simulink model "ADMIRE"  (R2021b)
settings: Solver=ode4  StartTime=0.0  StopTime=100  FixedStep=1e-2  RelTol=1e-3
undefined symbols (not defined in the file or in its folder): admireDB, Earth, WGS84
libraries: simulink_extras x112, simulink x27, aerolibutil x4, dspsigops x4, aerolibfltsims x3, sharedtransform x2, aerolibtransform2 x2, aerolibatmos2 x1, matrix_library x1, sharedutil x1, aerolibanimutils x1, vrlib x1
(part 10 of 15)

== system ADMIRE/Aircraft/Aerodynamics/CentripetalForceCoefficient/MachRegion2/Ccrbeta/Ccrbeta_ ==
  angleOfSideslip_deg : Inport
  angleOfAttack_deg : Inport  Port=2
  tflow : Inport  Port=3
  rc : Inport  Port=4
  Abs : Abs
  CCRBA_BETA_ALFA : Lookup_n-D  BreakpointsForDimension1=admireDB.aerodata_asym_ext.CCRBA.breakpoints.ALFA  BreakpointsForDimension2=admireDB.aerodata_asym_ext.CCRBA.breakpoints.BETA  BreakpointsForDimension3=[5, 7]  Table=admireDB.aerodata_asym_ext.CCRBA.newTable  ExtrapMethod=Clip  InternalRulePriority=Speed  RndMeth=Simplest  InputSameDT=on
      settings: InputPortMap=u0,u1
  Product : Product  Inputs=3
  Ccrbeta : Outport
  wires:
  Product/1 -> Ccrbeta/1
  rc/1 -> Product/3
  Abs/1 -> CCRBA_BETA_ALFA/2
  angleOfSideslip_deg/1 -> Abs/1
  angleOfAttack_deg/1 -> CCRBA_BETA_ALFA/1
  tflow/1 -> Product/2
  CCRBA_BETA_ALFA/1 -> Product/1

== system ADMIRE/Aircraft/Aerodynamics/CentripetalForceCoefficient/MachRegion3/Ccbcai/Ccbcai_ ==
  cai : Inport
  angleOfAttack_deg : Inport  Port=2
  angleOfSideslip_deg : Inport  Port=3
  CCBCAI_CAI_ALFA : Lookup_n-D  BreakpointsForDimension1=admireDB.aerodata_asym_ext.CCBCAI.breakpoints.ALFA  BreakpointsForDimension2=admireDB.aerodata_asym_ext.CCBCAI.breakpoints.CAI  BreakpointsForDimension3=[5, 7]  Table=admireDB.aerodata_asym_ext.CCBCAI.newTable  ExtrapMethod=Clip  InternalRulePriority=Speed  RndMeth=Simplest  InputSameDT=on
      settings: InputPortMap=u0,u1
  Degrees to Radians : simulink_extras/Transformations/Degrees to Radians
  Product : Product
  Ccbcai : Outport
  wires:
  CCBCAI_CAI_ALFA/1 -> Product/1
  Degrees to Radians/1 -> Product/2
  angleOfSideslip_deg/1 -> Degrees to Radians/1
  angleOfAttack_deg/1 -> CCBCAI_CAI_ALFA/1
  cai/1 -> CCBCAI_CAI_ALFA/2
  Product/1 -> Ccbcai/1

== system ADMIRE/Aircraft/Aerodynamics/CentripetalForceCoefficient/MachRegion3/Ccbde/Ccbde_ ==
  angleOfAttack_deg : Inport
  dEI : Inport  Port=2
  angleOfSideslip_deg : Inport  Port=3
  dEY : Inport  Port=4
  eieff : Inport  Port=5
  eoeff : Inport  Port=6
  mach_nd : Inport  Port=7
  Abs : Abs
  CCBKM_M : Lookup_n-D  NumberOfTableDimensions=1  BreakpointsForDimension1=admireDB.aerodata_asym_ext.CCBKM.breakpoints.M  BreakpointsForDimension3=[5, 7]  Table=admireDB.aerodata_asym_ext.CCBKM.newTable  ExtrapMethod=Clip  InternalRulePriority=Speed  RndMeth=Simplest  InputSameDT=on
  CCDEB_ALFA_DE_BETA : Lookup_n-D  NumberOfTableDimensions=3  BreakpointsForDimension1=admireDB.aerodata_asym_ext.CCDEB.breakpoints.ALFA  BreakpointsForDimension2=admireDB.aerodata_asym_ext.CCDEB.breakpoints.DE  BreakpointsForDimension3=admireDB.aerodata_asym_ext.CCDEB.breakpoints.BETA  Table=admireDB.aerodata_asym_ext.CCDEB.newTable  ExtrapMethod=Clip  InternalRulePriority=Speed  RndMeth=Simplest  InputSameDT=on
      settings: InputPortMap=u0,u1,u2
  CCDEB_ALFA_DE_BETA1 : Lookup_n-D  NumberOfTableDimensions=3  BreakpointsForDimension1=admireDB.aerodata_asym_ext.CCDEB.breakpoints.ALFA  BreakpointsForDimension2=admireDB.aerodata_asym_ext.CCDEB.breakpoints.DE  BreakpointsForDimension3=admireDB.aerodata_asym_ext.CCDEB.breakpoints.BETA  Table=admireDB.aerodata_asym_ext.CCDEB.newTable  ExtrapMethod=Clip  InternalRulePriority=Speed  RndMeth=Simplest  InputSameDT=on
      settings: InputPortMap=u0,u1,u2
  Product : Product
  Product1 : Product
  Product2 : Product  Inputs=3
  Sign : Signum
  Sum : Sum  Inputs=|++
  Ccbde : Outport
  wires:
  mach_nd/1 -> CCBKM_M/1
  CCBKM_M/1 -> Product2/3
  Abs/1 -> CCDEB_ALFA_DE_BETA1/3, CCDEB_ALFA_DE_BETA/3
  angleOfSideslip_deg/1 -> Abs/1, Sign/1
  Sign/1 -> Product2/2
  Sum/1 -> Product2/1
  Product1/1 -> Sum/2
  Product/1 -> Sum/1
  CCDEB_ALFA_DE_BETA1/1 -> Product1/1
  eoeff/1 -> Product1/2
  dEY/1 -> CCDEB_ALFA_DE_BETA1/2
  CCDEB_ALFA_DE_BETA/1 -> Product/1
  eieff/1 -> Product/2
  dEI/1 -> CCDEB_ALFA_DE_BETA/2
  angleOfAttack_deg/1 -> CCDEB_ALFA_DE_BETA1/1, CCDEB_ALFA_DE_BETA/1
  Product2/1 -> Ccbde/1

== system ADMIRE/Aircraft/Aerodynamics/CentripetalForceCoefficient/MachRegion3/Ccbdle/Ccbdle_ ==
  mach_nd : Inport
  angleOfAttack_deg : Inport  Port=2
  angleOfSideslip_deg : Inport  Port=3
  dLE : Inport  Port=4
  CCBDLE_M_ALFA : Lookup_n-D  BreakpointsForDimension1=admireDB.aerodata_asym_ext.CCBDLE.breakpoints.ALFA  BreakpointsForDimension2=admireDB.aerodata_asym_ext.CCBDLE.breakpoints.M  BreakpointsForDimension3=[5, 7]  Table=admireDB.aerodata_asym_ext.CCBDLE.newTable  ExtrapMethod=Clip  InternalRulePriority=Speed  RndMeth=Simplest  InputSameDT=on
      settings: InputPortMap=u0,u1
  Constant1 : Constant  Value=1/27
  Degrees to Radians : simulink_extras/Transformations/Degrees to Radians
  Product1 : Product  Inputs=4
  Ccbdle : Outport
  wires:
  dLE/1 -> Product1/3
  Product1/1 -> Ccbdle/1
  Constant1/1 -> Product1/4
  CCBDLE_M_ALFA/1 -> Product1/1
  Degrees to Radians/1 -> Product1/2
  angleOfAttack_deg/1 -> CCBDLE_M_ALFA/1
  angleOfSideslip_deg/1 -> Degrees to Radians/1
  mach_nd/1 -> CCBDLE_M_ALFA/2

== system ADMIRE/Aircraft/Aerodynamics/CentripetalForceCoefficient/MachRegion3/Ccbdn/Ccbdn_ ==
  angleOfAttack_deg : Inport
  dN : Inport  Port=2
  angleOfSideslip_deg : Inport  Port=3
  Abs : Abs
  CCDNB_ALFA_DN_BETA : Lookup_n-D  NumberOfTableDimensions=3  BreakpointsForDimension1=admireDB.aerodata_asym_ext.CCDNB.breakpoints.ALFA  BreakpointsForDimension2=admireDB.aerodata_asym_ext.CCDNB.breakpoints.DN  BreakpointsForDimension3=admireDB.aerodata_asym_ext.CCDNB.breakpoints.BETA  Table=admireDB.aerodata_asym_ext.CCDNB.newTable  ExtrapMethod=Clip  InternalRulePriority=Speed  RndMeth=Simplest  InputSameDT=on
      settings: InputPortMap=u0,u1,u2
  Product : Product
  Sign : Signum
  Ccbdn : Outport
  wires:
  Product/1 -> Ccbdn/1
  Sign/1 -> Product/2
  CCDNB_ALFA_DN_BETA/1 -> Product/1
  Abs/1 -> CCDNB_ALFA_DN_BETA/3
  angleOfSideslip_deg/1 -> Abs/1, Sign/1
  dN/1 -> CCDNB_ALFA_DN_BETA/2
  angleOfAttack_deg/1 -> CCDNB_ALFA_DN_BETA/1

== system ADMIRE/Aircraft/Aerodynamics/CentripetalForceCoefficient/MachRegion3/Ccbeta/Ccbeta_ ==
  mach_nd : Inport
  angleOfAttack_deg : Inport  Port=2
  angleOfSideslip_deg : Inport  Port=3
  qacorr : Inport  Port=4
  CCBMA_M_ALFA : Lookup_n-D  BreakpointsForDimension1=admireDB.aerodata_asym_ext.CCBMA.breakpoints.ALFA  BreakpointsForDimension2=admireDB.aerodata_asym_ext.CCBMA.breakpoints.M  BreakpointsForDimension3=[5, 7]  Table=admireDB.aerodata_asym_ext.CCBMA.newTable  ExtrapMethod=Clip  InternalRulePriority=Speed  RndMeth=Simplest  InputSameDT=on
      settings: InputPortMap=u0,u1
  CCEB_QA_M : Lookup_n-D  BreakpointsForDimension1=admireDB.aerodata_asym_ext.CCEB.breakpoints.M  BreakpointsForDimension2=admireDB.aerodata_asym_ext.CCEB.breakpoints.QA  BreakpointsForDimension3=[5, 7]  Table=admireDB.aerodata_asym_ext.CCEB.newTable  ExtrapMethod=Clip  InternalRulePriority=Speed  RndMeth=Simplest  InputSameDT=on
      settings: InputPortMap=u0,u1
  Degrees to Radians : simulink_extras/Transformations/Degrees to Radians
  Product : Product  Inputs=3
  CCbeta : Outport
  wires:
  Product/1 -> CCbeta/1
  CCEB_QA_M/1 -> Product/3
  qacorr/1 -> CCEB_QA_M/2
  Degrees to Radians/1 -> Product/2
  mach_nd/1 -> CCBMA_M_ALFA/2, CCEB_QA_M/1
  CCBMA_M_ALFA/1 -> Product/1
  angleOfAttack_deg/1 -> CCBMA_M_ALFA/1
  angleOfSideslip_deg/1 -> Degrees to Radians/1

== system ADMIRE/Aircraft/Aerodynamics/CentripetalForceCoefficient/MachRegion3/Ccbetad/Ccbetad_ ==
  angleOfAttack_deg : Inport
  mach_nd : Inport  Port=2
  betad : Inport  Port=3
  CCBDH_ALFA_M : Lookup_n-D  BreakpointsForDimension1=admireDB.aerodata_asym_ext.CCBDH.breakpoints.M  BreakpointsForDimension2=admireDB.aerodata_asym_ext.CCBDH.breakpoints.ALFA  BreakpointsForDimension3=[5, 7]  Table=admireDB.aerodata_asym_ext.CCBDH.newTable  ExtrapMethod=Clip  InternalRulePriority=Speed  RndMeth=Simplest  InputSameDT=on
      settings: InputPortMap=u0,u1
  Product1 : Product
  CCbetad : Outport
  wires:
  betad/1 -> Product1/2
  mach_nd/1 -> CCBDH_ALFA_M/1
  CCBDH_ALFA_M/1 -> Product1/1
  angleOfAttack_deg/1 -> CCBDH_ALFA_M/2
  Product1/1 -> CCbetad/1

== system ADMIRE/Aircraft/Aerodynamics/CentripetalForceCoefficient/MachRegion3/Ccblg/Ccblg_ ==
  ldg : Inport
  angleOfAttack_deg : Inport  Port=2
  angleOfSideslip_deg : Inport  Port=3
  CCBLST_NG_DOOR_ALFA : Lookup_n-D  BreakpointsForDimension1=admireDB.aerodata_asym_ext.CCBLST.breakpoints.ALFA  BreakpointsForDimension2=admireDB.aerodata_asym_ext.CCBLST.breakpoints.NG_DOOR  BreakpointsForDimension3=[5, 7]  Table=admireDB.aerodata_asym_ext.CCBLST.newTable  ExtrapMethod=Clip  InternalRulePriority=Speed  RndMeth=Simplest  InputSameDT=on
      settings: InputPortMap=u0,u1
  Degrees to Radians : simulink_extras/Transformations/Degrees to Radians
  Product : Product  Inputs=3
  Ccblg : Outport
  wires:
  Degrees to Radians/1 -> Product/3
  CCBLST_NG_DOOR_ALFA/1 -> Product/2
  angleOfSideslip_deg/1 -> Degrees to Radians/1
  ldg/1 -> CCBLST_NG_DOOR_ALFA/2, Product/1
  angleOfAttack_deg/1 -> CCBLST_NG_DOOR_ALFA/1
  Product/1 -> Ccblg/1

== system ADMIRE/Aircraft/Aerodynamics/CentripetalForceCoefficient/MachRegion3/Ccdai/Ccdai_ ==
  angleOfAttack_deg : Inport
  dAI : Inport  Port=2
  mach_nd : Inport  Port=3
  dEI : Inport  Port=4
  eieff : Inport  Port=5
  qacorr : Inport  Port=6
  Abs : Abs
  CCDA_ALFA_DE_M : Lookup_n-D  NumberOfTableDimensions=3  BreakpointsForDimension1=admireDB.aerodata_asym_ext.CCDA.breakpoints.ALFA  BreakpointsForDimension2=admireDB.aerodata_asym_ext.CCDA.breakpoints.DE  BreakpointsForDimension3=admireDB.aerodata_asym_ext.CCDA.breakpoints.M  Table=admireDB.aerodata_asym_ext.CCDA.newTable  ExtrapMethod=Clip  InternalRulePriority=Speed  RndMeth=Simplest  InputSameDT=on
      settings: InputPortMap=u0,u1,u2
  CCDA_ALFA_DE_M1 : Lookup_n-D  NumberOfTableDimensions=3  BreakpointsForDimension1=admireDB.aerodata_asym_ext.CCDA.breakpoints.ALFA  BreakpointsForDimension2=admireDB.aerodata_asym_ext.CCDA.breakpoints.DE  BreakpointsForDimension3=admireDB.aerodata_asym_ext.CCDA.breakpoints.M  Table=admireDB.aerodata_asym_ext.CCDA.newTable  ExtrapMethod=Clip  InternalRulePriority=Speed  RndMeth=Simplest  InputSameDT=on
      settings: InputPortMap=u0,u1,u2
  CCEDAI_QA_M : Lookup_n-D  BreakpointsForDimension1=admireDB.aerodata_asym_ext.CCEDAI.breakpoints.M  BreakpointsForDimension2=admireDB.aerodata_asym_ext.CCEDAI.breakpoints.QA  BreakpointsForDimension3=[5, 7]  Table=admireDB.aerodata_asym_ext.CCEDAI.newTable  ExtrapMethod=Clip  InternalRulePriority=Speed  RndMeth=Simplest  InputSameDT=on
      settings: InputPortMap=u0,u1
  CCMDAA_ALFA_DA_M : Lookup_n-D  NumberOfTableDimensions=3  BreakpointsForDimension1=admireDB.aerodata_asym_ext.CCMDAA.breakpoints.ALFA  BreakpointsForDimension2=admireDB.aerodata_asym_ext.CCMDAA.breakpoints.DA  BreakpointsForDimension3=admireDB.aerodata_asym_ext.CCMDAA.breakpoints.M  Table=admireDB.aerodata_asym_ext.CCMDAA.newTable  ExtrapMethod=Clip  InternalRulePriority=Speed  RndMeth=Simplest  InputSameDT=on
      settings: InputPortMap=u0,u1,u2
  Constant : Constant  Value=0
  Degrees to Radians : simulink_extras/Transformations/Degrees to Radians
  Product : Product
  Product1 : Product
  Product2 : Product  Inputs=3
  Sign : Signum
  Sum : Sum  Inputs=|+-
  Sum1 : Sum  Inputs=|++
  Ccdai : Outport
  wires:
  CCDA_ALFA_DE_M1/1 -> Sum/2
  CCEDAI_QA_M/1 -> Product2/3
  qacorr/1 -> CCEDAI_QA_M/2
  Product2/1 -> Ccdai/1
  eieff/1 -> Product2/2
  Sum1/1 -> Product2/1
  Product1/1 -> Sum1/2
  Product/1 -> Sum1/1
  dEI/1 -> CCDA_ALFA_DE_M/2
  Constant/1 -> CCDA_ALFA_DE_M1/2
  Sum/1 -> Product1/2
  CCDA_ALFA_DE_M/1 -> Sum/1
  Degrees to Radians/1 -> Product1/1
  CCMDAA_ALFA_DA_M/1 -> Product/1
  Sign/1 -> Product/2
  mach_nd/1 -> CCDA_ALFA_DE_M1/3, CCEDAI_QA_M/1, CCDA_ALFA_DE_M/3, CCMDAA_ALFA_DA_M/3
  Abs/1 -> CCMDAA_ALFA_DA_M/2
  angleOfAttack_deg/1 -> CCDA_ALFA_DE_M1/1, CCDA_ALFA_DE_M/1, CCMDAA_ALFA_DA_M/1
  dAI/1 -> Abs/1, Sign/1, Degrees to Radians/1

== system ADMIRE/Aircraft/Aerodynamics/CentripetalForceCoefficient/MachRegion3/Ccday/Ccday_ ==
  angleOfAttack_deg : Inport
  dAY : Inport  Port=2
  mach_nd : Inport  Port=3
  dEY : Inport  Port=4
  eoeff : Inport  Port=5
  qacorr : Inport  Port=6
  Abs : Abs
  CCDA_ALFA_DE_M : Lookup_n-D  NumberOfTableDimensions=3  BreakpointsForDimension1=admireDB.aerodata_asym_ext.CCDA.breakpoints.ALFA  BreakpointsForDimension2=admireDB.aerodata_asym_ext.CCDA.breakpoints.DE  BreakpointsForDimension3=admireDB.aerodata_asym_ext.CCDA.breakpoints.M  Table=admireDB.aerodata_asym_ext.CCDA.newTable  ExtrapMethod=Clip  InternalRulePriority=Speed  RndMeth=Simplest  InputSameDT=on
      settings: InputPortMap=u0,u1,u2
  CCDA_ALFA_DE_M1 : Lookup_n-D  NumberOfTableDimensions=3  BreakpointsForDimension1=admireDB.aerodata_asym_ext.CCDA.breakpoints.ALFA  BreakpointsForDimension2=admireDB.aerodata_asym_ext.CCDA.breakpoints.DE  BreakpointsForDimension3=admireDB.aerodata_asym_ext.CCDA.breakpoints.M  Table=admireDB.aerodata_asym_ext.CCDA.newTable  ExtrapMethod=Clip  InternalRulePriority=Speed  RndMeth=Simplest  InputSameDT=on
      settings: InputPortMap=u0,u1,u2
  CCEDAY_QA_M : Lookup_n-D  BreakpointsForDimension1=admireDB.aerodata_asym_ext.CCEDAY.breakpoints.M  BreakpointsForDimension2=admireDB.aerodata_asym_ext.CCEDAY.breakpoints.QA  BreakpointsForDimension3=[5, 7]  Table=admireDB.aerodata_asym_ext.CCEDAY.newTable  ExtrapMethod=Clip  InternalRulePriority=Speed  RndMeth=Simplest  InputSameDT=on
      settings: InputPortMap=u0,u1
  CCMDAA_ALFA_DA_M : Lookup_n-D  NumberOfTableDimensions=3  BreakpointsForDimension1=admireDB.aerodata_asym_ext.CCMDAA.breakpoints.ALFA  BreakpointsForDimension2=admireDB.aerodata_asym_ext.CCMDAA.breakpoints.DA  BreakpointsForDimension3=admireDB.aerodata_asym_ext.CCMDAA.breakpoints.M  Table=admireDB.aerodata_asym_ext.CCMDAA.newTable  ExtrapMethod=Clip  InternalRulePriority=Speed  RndMeth=Simplest  InputSameDT=on
      settings: InputPortMap=u0,u1,u2
  Constant : Constant  Value=0
  Degrees to Radians : simulink_extras/Transformations/Degrees to Radians
  Product{,1..3} (4 alike) : Product
  Sign : Signum
  Sum : Sum  Inputs=|+-
  Sum1 : Sum  Inputs=|++
  Sum2 : Sum  Inputs=|++
  Ccday : Outport
  wires:
  Product3/1 -> Sum2/2
  Sum2/1 -> Ccday/1
  CCDA_ALFA_DE_M1/1 -> Sum/2
  CCEDAY_QA_M/1 -> Product3/2
  qacorr/1 -> CCEDAY_QA_M/2
  Product2/1 -> Sum2/1
  eoeff/1 -> Product2/2
  Sum1/1 -> Product2/1
  Product1/1 -> Sum1/2
  Product/1 -> Sum1/1
  dEY/1 -> CCDA_ALFA_DE_M/2
  Constant/1 -> CCDA_ALFA_DE_M1/2
  Sum/1 -> Product1/2
  CCDA_ALFA_DE_M/1 -> Sum/1
  Degrees to Radians/1 -> Product1/1, Product3/1
  CCMDAA_ALFA_DA_M/1 -> Product/1
  Sign/1 -> Product/2
  mach_nd/1 -> CCDA_ALFA_DE_M1/3, CCEDAY_QA_M/1, CCDA_ALFA_DE_M/3, CCMDAA_ALFA_DA_M/3
  Abs/1 -> CCMDAA_ALFA_DA_M/2
  angleOfAttack_deg/1 -> CCDA_ALFA_DE_M1/1, CCDA_ALFA_DE_M/1, CCMDAA_ALFA_DA_M/1
  dAY/1 -> Abs/1, Sign/1, Degrees to Radians/1

== system ADMIRE/Aircraft/Aerodynamics/CentripetalForceCoefficient/MachRegion3/Ccdna/Ccdna_ ==
  angleOfAttack_deg : Inport
  mach_nd : Inport  Port=2
  dNA : Inport  Port=3
  CCDNAAM_ALFA_M : Lookup_n-D  BreakpointsForDimension1=admireDB.aerodata_asym_ext.CCDNAAM.breakpoints.M  BreakpointsForDimension2=admireDB.aerodata_asym_ext.CCDNAAM.breakpoints.ALFA  BreakpointsForDimension3=[5, 7]  Table=admireDB.aerodata_asym_ext.CCDNAAM.newTable  ExtrapMethod=Clip  InternalRulePriority=Speed  RndMeth=Simplest  InputSameDT=on
      settings: InputPortMap=u0,u1
  Degrees to Radians : simulink_extras/Transformations/Degrees to Radians
  Product1 : Product
  Ccdna : Outport
  wires:
  Degrees to Radians/1 -> Product1/2
  dNA/1 -> Degrees to Radians/1
  Product1/1 -> Ccdna/1
  mach_nd/1 -> CCDNAAM_ALFA_M/1
  CCDNAAM_ALFA_M/1 -> Product1/1
  angleOfAttack_deg/1 -> CCDNAAM_ALFA_M/2

== system ADMIRE/Aircraft/Aerodynamics/CentripetalForceCoefficient/MachRegion3/Ccdr/Ccdr_ ==
  angleOfAttack_deg : Inport
  mach_nd : Inport  Port=2
  dR : Inport  Port=3
  qacorr : Inport  Port=4
  CCDRAM_ALFA_M : Lookup_n-D  BreakpointsForDimension1=admireDB.aerodata_asym_ext.CCDRAM.breakpoints.M  BreakpointsForDimension2=admireDB.aerodata_asym_ext.CCDRAM.breakpoints.ALFA  BreakpointsForDimension3=[5, 7]  Table=admireDB.aerodata_asym_ext.CCDRAM.newTable  ExtrapMethod=Clip  InternalRulePriority=Speed  RndMeth=Simplest  InputSameDT=on
      settings: InputPortMap=u0,u1
  CCEDR_QA_M : Lookup_n-D  BreakpointsForDimension1=admireDB.aerodata_asym_ext.CCEDR.breakpoints.M  BreakpointsForDimension2=admireDB.aerodata_asym_ext.CCEDR.breakpoints.QA  BreakpointsForDimension3=[5, 7]  Table=admireDB.aerodata_asym_ext.CCEDR.newTable  ExtrapMethod=Clip  InternalRulePriority=Speed  RndMeth=Simplest  InputSameDT=on
      settings: InputPortMap=u0,u1
  Degrees to Radians : simulink_extras/Transformations/Degrees to Radians
  Product1 : Product  Inputs=3
  Ccdr : Outport
  wires:
  CCEDR_QA_M/1 -> Product1/3
  Product1/1 -> Ccdr/1
  mach_nd/1 -> CCDRAM_ALFA_M/1, CCEDR_QA_M/1
  qacorr/1 -> CCEDR_QA_M/2
  Degrees to Radians/1 -> Product1/2
  CCDRAM_ALFA_M/1 -> Product1/1
  dR/1 -> Degrees to Radians/1
  angleOfAttack_deg/1 -> CCDRAM_ALFA_M/2

== system ADMIRE/Aircraft/Aerodynamics/CentripetalForceCoefficient/MachRegion3/Ccp1/Ccp_ ==
  angleOfAttack_deg : Inport
  mach_nd : Inport  Port=2
  pc : Inport  Port=3
  CCPAM_ALFA_M : Lookup_n-D  BreakpointsForDimension1=admireDB.aerodata_asym_ext.CCPAM.breakpoints.M  BreakpointsForDimension2=admireDB.aerodata_asym_ext.CCPAM.breakpoints.ALFA  BreakpointsForDimension3=[5, 7]  Table=admireDB.aerodata_asym_ext.CCPAM.newTable  ExtrapMethod=Clip  InternalRulePriority=Speed  RndMeth=Simplest  InputSameDT=on
      settings: InputPortMap=u0,u1
  Product2 : Product
  Ccp : Outport
  wires:
  mach_nd/1 -> CCPAM_ALFA_M/1
  CCPAM_ALFA_M/1 -> Product2/1
  Product2/1 -> Ccp/1
  pc/1 -> Product2/2
  angleOfAttack_deg/1 -> CCPAM_ALFA_M/2

== system ADMIRE/Aircraft/Aerodynamics/CentripetalForceCoefficient/MachRegion3/Ccr1/Ccr_ ==
  mach_nd : Inport
  rc : Inport  Port=2
  CCRM_M : Lookup_n-D  NumberOfTableDimensions=1  BreakpointsForDimension1=admireDB.aerodata_asym_ext.CCRM.breakpoints.M  BreakpointsForDimension3=[5, 7]  Table=admireDB.aerodata_asym_ext.CCRM.newTable  ExtrapMethod=Clip  InternalRulePriority=Speed  RndMeth=Simplest  InputSameDT=on
  Product2 : Product
  Ccr : Outport
  wires:
  Product2/1 -> Ccr/1
  CCRM_M/1 -> Product2/1
  mach_nd/1 -> CCRM_M/1
  rc/1 -> Product2/2

== system ADMIRE/Aircraft/Aerodynamics/CentripetalForceCoefficient/MachRegion4/Ccbcai/Ccbcai_ ==
  cai : Inport
  angleOfAttack_deg : Inport  Port=2
  angleOfSideslip_deg : Inport  Port=3
  CCBCAI_CAI_ALFA : Lookup_n-D  BreakpointsForDimension1=admireDB.aerodata_asym_ext.CCBCAI.breakpoints.ALFA  BreakpointsForDimension2=admireDB.aerodata_asym_ext.CCBCAI.breakpoints.CAI  BreakpointsForDimension3=[5, 7]  Table=admireDB.aerodata_asym_ext.CCBCAI.newTable  ExtrapMethod=Clip  InternalRulePriority=Speed  RndMeth=Simplest  InputSameDT=on
      settings: InputPortMap=u0,u1
  Degrees to Radians : simulink_extras/Transformations/Degrees to Radians
  Product : Product
  Ccbcai : Outport
  wires:
  CCBCAI_CAI_ALFA/1 -> Product/1
  Degrees to Radians/1 -> Product/2
  angleOfSideslip_deg/1 -> Degrees to Radians/1
  angleOfAttack_deg/1 -> CCBCAI_CAI_ALFA/1
  cai/1 -> CCBCAI_CAI_ALFA/2
  Product/1 -> Ccbcai/1

== system ADMIRE/Aircraft/Aerodynamics/CentripetalForceCoefficient/MachRegion4/Ccbde/Ccbde_ ==
  angleOfAttack_deg : Inport
  dEI : Inport  Port=2
  angleOfSideslip_deg : Inport  Port=3
  dEY : Inport  Port=4
  eieff : Inport  Port=5
  eoeff : Inport  Port=6
  mach_nd : Inport  Port=7
  Abs : Abs
  CCBKM_M : Lookup_n-D  NumberOfTableDimensions=1  BreakpointsForDimension1=admireDB.aerodata_asym_ext.CCBKM.breakpoints.M  BreakpointsForDimension3=[5, 7]  Table=admireDB.aerodata_asym_ext.CCBKM.newTable  ExtrapMethod=Clip  InternalRulePriority=Speed  RndMeth=Simplest  InputSameDT=on
  CCDEB_ALFA_DE_BETA : Lookup_n-D  NumberOfTableDimensions=3  BreakpointsForDimension1=admireDB.aerodata_asym_ext.CCDEB.breakpoints.ALFA  BreakpointsForDimension2=admireDB.aerodata_asym_ext.CCDEB.breakpoints.DE  BreakpointsForDimension3=admireDB.aerodata_asym_ext.CCDEB.breakpoints.BETA  Table=admireDB.aerodata_asym_ext.CCDEB.newTable  ExtrapMethod=Clip  InternalRulePriority=Speed  RndMeth=Simplest  InputSameDT=on
      settings: InputPortMap=u0,u1,u2
  CCDEB_ALFA_DE_BETA1 : Lookup_n-D  NumberOfTableDimensions=3  BreakpointsForDimension1=admireDB.aerodata_asym_ext.CCDEB.breakpoints.ALFA  BreakpointsForDimension2=admireDB.aerodata_asym_ext.CCDEB.breakpoints.DE  BreakpointsForDimension3=admireDB.aerodata_asym_ext.CCDEB.breakpoints.BETA  Table=admireDB.aerodata_asym_ext.CCDEB.newTable  ExtrapMethod=Clip  InternalRulePriority=Speed  RndMeth=Simplest  InputSameDT=on
      settings: InputPortMap=u0,u1,u2
  Product : Product
  Product1 : Product
  Product2 : Product  Inputs=3
  Sign : Signum
  Sum : Sum  Inputs=|++
  Ccbde : Outport
  wires:
  mach_nd/1 -> CCBKM_M/1
  CCBKM_M/1 -> Product2/3
  Abs/1 -> CCDEB_ALFA_DE_BETA1/3, CCDEB_ALFA_DE_BETA/3
  angleOfSideslip_deg/1 -> Abs/1, Sign/1
  Sign/1 -> Product2/2
  Sum/1 -> Product2/1
  Product1/1 -> Sum/2
  Product/1 -> Sum/1
  CCDEB_ALFA_DE_BETA1/1 -> Product1/1
  eoeff/1 -> Product1/2
  dEY/1 -> CCDEB_ALFA_DE_BETA1/2
  CCDEB_ALFA_DE_BETA/1 -> Product/1
  eieff/1 -> Product/2
  dEI/1 -> CCDEB_ALFA_DE_BETA/2
  angleOfAttack_deg/1 -> CCDEB_ALFA_DE_BETA1/1, CCDEB_ALFA_DE_BETA/1
  Product2/1 -> Ccbde/1

== system ADMIRE/Aircraft/Aerodynamics/CentripetalForceCoefficient/MachRegion4/Ccbdle/Ccbdle_ ==
  mach_nd : Inport
  angleOfAttack_deg : Inport  Port=2
  angleOfSideslip_deg : Inport  Port=3
  dLE : Inport  Port=4
  CCBDLE_M_ALFA : Lookup_n-D  BreakpointsForDimension1=admireDB.aerodata_asym_ext.CCBDLE.breakpoints.ALFA  BreakpointsForDimension2=admireDB.aerodata_asym_ext.CCBDLE.breakpoints.M  BreakpointsForDimension3=[5, 7]  Table=admireDB.aerodata_asym_ext.CCBDLE.newTable  ExtrapMethod=Clip  InternalRulePriority=Speed  RndMeth=Simplest  InputSameDT=on
      settings: InputPortMap=u0,u1
  Constant1 : Constant  Value=1/27
  Degrees to Radians : simulink_extras/Transformations/Degrees to Radians
  Product1 : Product  Inputs=4
  Ccbdle : Outport
  wires:
  dLE/1 -> Product1/3
  Product1/1 -> Ccbdle/1
  Constant1/1 -> Product1/4
  CCBDLE_M_ALFA/1 -> Product1/1
  Degrees to Radians/1 -> Product1/2
  angleOfAttack_deg/1 -> CCBDLE_M_ALFA/1
  angleOfSideslip_deg/1 -> Degrees to Radians/1
  mach_nd/1 -> CCBDLE_M_ALFA/2

== system ADMIRE/Aircraft/Aerodynamics/CentripetalForceCoefficient/MachRegion4/Ccbdn/Ccbdn_ ==
  angleOfAttack_deg : Inport
  dN : Inport  Port=2
  angleOfSideslip_deg : Inport  Port=3
  Abs : Abs
  CCDNB_ALFA_DN_BETA : Lookup_n-D  NumberOfTableDimensions=3  BreakpointsForDimension1=admireDB.aerodata_asym_ext.CCDNB.breakpoints.ALFA  BreakpointsForDimension2=admireDB.aerodata_asym_ext.CCDNB.breakpoints.DN  BreakpointsForDimension3=admireDB.aerodata_asym_ext.CCDNB.breakpoints.BETA  Table=admireDB.aerodata_asym_ext.CCDNB.newTable  ExtrapMethod=Clip  InternalRulePriority=Speed  RndMeth=Simplest  InputSameDT=on
      settings: InputPortMap=u0,u1,u2
  Product : Product
  Sign : Signum
  Ccbdn : Outport
  wires:
  Product/1 -> Ccbdn/1
  Sign/1 -> Product/2
  CCDNB_ALFA_DN_BETA/1 -> Product/1
  Abs/1 -> CCDNB_ALFA_DN_BETA/3
  angleOfSideslip_deg/1 -> Abs/1, Sign/1
  dN/1 -> CCDNB_ALFA_DN_BETA/2
  angleOfAttack_deg/1 -> CCDNB_ALFA_DN_BETA/1

== system ADMIRE/Aircraft/Aerodynamics/CentripetalForceCoefficient/MachRegion4/Ccbeta/Ccbeta_ ==
  mach_nd : Inport
  angleOfAttack_deg : Inport  Port=2
  angleOfSideslip_deg : Inport  Port=3
  qacorr : Inport  Port=4
  CCBMA_M_ALFA : Lookup_n-D  BreakpointsForDimension1=admireDB.aerodata_asym_ext.CCBMA.breakpoints.ALFA  BreakpointsForDimension2=admireDB.aerodata_asym_ext.CCBMA.breakpoints.M  BreakpointsForDimension3=[5, 7]  Table=admireDB.aerodata_asym_ext.CCBMA.newTable  ExtrapMethod=Clip  InternalRulePriority=Speed  RndMeth=Simplest  InputSameDT=on
      settings: InputPortMap=u0,u1
  CCEB_QA_M : Lookup_n-D  BreakpointsForDimension1=admireDB.aerodata_asym_ext.CCEB.breakpoints.M  BreakpointsForDimension2=admireDB.aerodata_asym_ext.CCEB.breakpoints.QA  BreakpointsForDimension3=[5, 7]  Table=admireDB.aerodata_asym_ext.CCEB.newTable  ExtrapMethod=Clip  InternalRulePriority=Speed  RndMeth=Simplest  InputSameDT=on
      settings: InputPortMap=u0,u1
  Degrees to Radians : simulink_extras/Transformations/Degrees to Radians
  Product : Product  Inputs=3
  CCbeta : Outport
  wires:
  angleOfSideslip_deg/1 -> Degrees to Radians/1
  angleOfAttack_deg/1 -> CCBMA_M_ALFA/1
  CCBMA_M_ALFA/1 -> Product/1  "CCBAL"
  mach_nd/1 -> CCBMA_M_ALFA/2, CCEB_QA_M/1
  Degrees to Radians/1 -> Product/2
  qacorr/1 -> CCEB_QA_M/2
  CCEB_QA_M/1 -> Product/3
  Product/1 -> CCbeta/1

== system ADMIRE/Aircraft/Aerodynamics/CentripetalForceCoefficient/MachRegion4/Ccbetad/Ccbetad_ ==
  angleOfAttack_deg : Inport
  mach_nd : Inport  Port=2
  betad : Inport  Port=3
  CCBDH_ALFA_M : Lookup_n-D  BreakpointsForDimension1=admireDB.aerodata_asym_ext.CCBDH.breakpoints.M  BreakpointsForDimension2=admireDB.aerodata_asym_ext.CCBDH.breakpoints.ALFA  BreakpointsForDimension3=[5, 7]  Table=admireDB.aerodata_asym_ext.CCBDH.newTable  ExtrapMethod=Clip  InternalRulePriority=Speed  RndMeth=Simplest  InputSameDT=on
      settings: InputPortMap=u0,u1
  Product1 : Product
  CCbetad : Outport
  wires:
  betad/1 -> Product1/2
  mach_nd/1 -> CCBDH_ALFA_M/1
  CCBDH_ALFA_M/1 -> Product1/1
  angleOfAttack_deg/1 -> CCBDH_ALFA_M/2
  Product1/1 -> CCbetad/1

== system ADMIRE/Aircraft/Aerodynamics/CentripetalForceCoefficient/MachRegion4/Ccblg/Ccblg_ ==
  ldg : Inport
  angleOfAttack_deg : Inport  Port=2
  angleOfSideslip_deg : Inport  Port=3
  CCBLST_NG_DOOR_ALFA : Lookup_n-D  BreakpointsForDimension1=admireDB.aerodata_asym_ext.CCBLST.breakpoints.ALFA  BreakpointsForDimension2=admireDB.aerodata_asym_ext.CCBLST.breakpoints.NG_DOOR  BreakpointsForDimension3=[5, 7]  Table=admireDB.aerodata_asym_ext.CCBLST.newTable  ExtrapMethod=Clip  InternalRulePriority=Speed  RndMeth=Simplest  InputSameDT=on
      settings: InputPortMap=u0,u1
  Degrees to Radians : simulink_extras/Transformations/Degrees to Radians
  Product : Product  Inputs=3
  Ccblg : Outport
  wires:
  Degrees to Radians/1 -> Product/3
  CCBLST_NG_DOOR_ALFA/1 -> Product/2
  angleOfSideslip_deg/1 -> Degrees to Radians/1
  ldg/1 -> CCBLST_NG_DOOR_ALFA/2, Product/1
  angleOfAttack_deg/1 -> CCBLST_NG_DOOR_ALFA/1
  Product/1 -> Ccblg/1

== system ADMIRE/Aircraft/Aerodynamics/CentripetalForceCoefficient/MachRegion4/Ccdai/Ccdai_ ==
  dAI : Inport
  angleOfAttack_deg : Inport  Port=2
  dEI : Inport  Port=3
  qacorr : Inport  Port=4
  eieff : Inport  Port=5
  mach_nd : Inport  Port=6
  CCDA_ALFA_DE_M : Lookup_n-D  NumberOfTableDimensions=3  BreakpointsForDimension1=admireDB.aerodata_asym_ext.CCDA.breakpoints.ALFA  BreakpointsForDimension2=admireDB.aerodata_asym_ext.CCDA.breakpoints.DE  BreakpointsForDimension3=admireDB.aerodata_asym_ext.CCDA.breakpoints.M  Table=admireDB.aerodata_asym_ext.CCDA.newTable  ExtrapMethod=Clip  InternalRulePriority=Speed  RndMeth=Simplest  InputSameDT=on
      settings: InputPortMap=u0,u1,u2
  CCEDAI_QA_M : Lookup_n-D  BreakpointsForDimension1=admireDB.aerodata_asym_ext.CCEDAI.breakpoints.M  BreakpointsForDimension2=admireDB.aerodata_asym_ext.CCEDAI.breakpoints.QA  BreakpointsForDimension3=[5, 7]  Table=admireDB.aerodata_asym_ext.CCEDAI.newTable  ExtrapMethod=Clip  InternalRulePriority=Speed  RndMeth=Simplest  InputSameDT=on
      settings: InputPortMap=u0,u1
  Degrees to Radians : simulink_extras/Transformations/Degrees to Radians
  Product1 : Product  Inputs=4
  Ccdai : Outport
  wires:
  Product1/1 -> Ccdai/1
  eieff/1 -> Product1/2
  CCEDAI_QA_M/1 -> Product1/4
  qacorr/1 -> CCEDAI_QA_M/2
  dEI/1 -> CCDA_ALFA_DE_M/2
  CCDA_ALFA_DE_M/1 -> Product1/3
  Degrees to Radians/1 -> Product1/1
  mach_nd/1 -> CCDA_ALFA_DE_M/3, CCEDAI_QA_M/1
  angleOfAttack_deg/1 -> CCDA_ALFA_DE_M/1
  dAI/1 -> Degrees to Radians/1

== system ADMIRE/Aircraft/Aerodynamics/CentripetalForceCoefficient/MachRegion4/Ccday/Ccday_ ==
  angleOfAttack_deg : Inport
  dEY : Inport  Port=2
  mach_nd : Inport  Port=3
  qacorr : Inport  Port=4
  eoeff : Inport  Port=5
  dAY : Inport  Port=6
  CCDA_ALFA_DE_M : Lookup_n-D  NumberOfTableDimensions=3  BreakpointsForDimension1=admireDB.aerodata_asym_ext.CCDA.breakpoints.ALFA  BreakpointsForDimension2=admireDB.aerodata_asym_ext.CCDA.breakpoints.DE  BreakpointsForDimension3=admireDB.aerodata_asym_ext.CCDA.breakpoints.M  Table=admireDB.aerodata_asym_ext.CCDA.newTable  ExtrapMethod=Clip  InternalRulePriority=Speed  RndMeth=Simplest  InputSameDT=on
      settings: InputPortMap=u0,u1,u2
  CCEDAY_QA_M : Lookup_n-D  BreakpointsForDimension1=admireDB.aerodata_asym_ext.CCEDAY.breakpoints.M  BreakpointsForDimension2=admireDB.aerodata_asym_ext.CCEDAY.breakpoints.QA  BreakpointsForDimension3=[5, 7]  Table=admireDB.aerodata_asym_ext.CCEDAY.newTable  ExtrapMethod=Clip  InternalRulePriority=Speed  RndMeth=Simplest  InputSameDT=on
      settings: InputPortMap=u0,u1
  Degrees to Radians : simulink_extras/Transformations/Degrees to Radians
  Product : Product
  Product1 : Product
  Sum : Sum  Inputs=|++
  Ccday : Outport
  wires:
  Product1/1 -> Ccday/1
  dAY/1 -> Degrees to Radians/1
  Degrees to Radians/1 -> Product1/2
  Sum/1 -> Product1/1
  qacorr/1 -> CCEDAY_QA_M/2
  CCEDAY_QA_M/1 -> Sum/2
  Product/1 -> Sum/1
  CCDA_ALFA_DE_M/1 -> Product/1
  eoeff/1 -> Product/2
  mach_nd/1 -> CCDA_ALFA_DE_M/3, CCEDAY_QA_M/1
  dEY/1 -> CCDA_ALFA_DE_M/2
  angleOfAttack_deg/1 -> CCDA_ALFA_DE_M/1

== system ADMIRE/Aircraft/Aerodynamics/CentripetalForceCoefficient/MachRegion4/Ccdna/Ccdna_ ==
  angleOfAttack_deg : Inport
  mach_nd : Inport  Port=2
  dNA : Inport  Port=3
  CCDNAAM_ALFA_M : Lookup_n-D  BreakpointsForDimension1=admireDB.aerodata_asym_ext.CCDNAAM.breakpoints.M  BreakpointsForDimension2=admireDB.aerodata_asym_ext.CCDNAAM.breakpoints.ALFA  BreakpointsForDimension3=[5, 7]  Table=admireDB.aerodata_asym_ext.CCDNAAM.newTable  ExtrapMethod=Clip  InternalRulePriority=Speed  RndMeth=Simplest  InputSameDT=on
      settings: InputPortMap=u0,u1
  Degrees to Radians : simulink_extras/Transformations/Degrees to Radians
  Product1 : Product
  Ccdna : Outport
  wires:
  Degrees to Radians/1 -> Product1/2
  dNA/1 -> Degrees to Radians/1
  Product1/1 -> Ccdna/1
  mach_nd/1 -> CCDNAAM_ALFA_M/1
  CCDNAAM_ALFA_M/1 -> Product1/1
  angleOfAttack_deg/1 -> CCDNAAM_ALFA_M/2

== system ADMIRE/Aircraft/Aerodynamics/CentripetalForceCoefficient/MachRegion4/Ccdr/Ccdr_ ==
  angleOfAttack_deg : Inport
  mach_nd : Inport  Port=2
  dR : Inport  Port=3
  qacorr : Inport  Port=4
  CCDRAM_ALFA_M : Lookup_n-D  BreakpointsForDimension1=admireDB.aerodata_asym_ext.CCDRAM.breakpoints.M  BreakpointsForDimension2=admireDB.aerodata_asym_ext.CCDRAM.breakpoints.ALFA  BreakpointsForDimension3=[5, 7]  Table=admireDB.aerodata_asym_ext.CCDRAM.newTable  ExtrapMethod=Clip  InternalRulePriority=Speed  RndMeth=Simplest  InputSameDT=on
      settings: InputPortMap=u0,u1
  CCEDR_QA_M : Lookup_n-D  BreakpointsForDimension1=admireDB.aerodata_asym_ext.CCEDR.breakpoints.M  BreakpointsForDimension2=admireDB.aerodata_asym_ext.CCEDR.breakpoints.QA  BreakpointsForDimension3=[5, 7]  Table=admireDB.aerodata_asym_ext.CCEDR.newTable  ExtrapMethod=Clip  InternalRulePriority=Speed  RndMeth=Simplest  InputSameDT=on
      settings: InputPortMap=u0,u1
  Degrees to Radians : simulink_extras/Transformations/Degrees to Radians
  Product1 : Product  Inputs=3
  Ccdr : Outport
  wires:
  CCEDR_QA_M/1 -> Product1/3
  Product1/1 -> Ccdr/1
  mach_nd/1 -> CCEDR_QA_M/1, CCDRAM_ALFA_M/1
  qacorr/1 -> CCEDR_QA_M/2
  Degrees to Radians/1 -> Product1/2
  CCDRAM_ALFA_M/1 -> Product1/1
  dR/1 -> Degrees to Radians/1
  angleOfAttack_deg/1 -> CCDRAM_ALFA_M/2

== system ADMIRE/Aircraft/Aerodynamics/CentripetalForceCoefficient/MachRegion4/Ccp/Ccp_ ==
  angleOfAttack_deg : Inport
  mach_nd : Inport  Port=2
  pc : Inport  Port=3
  CCPAM_ALFA_M : Lookup_n-D  BreakpointsForDimension1=admireDB.aerodata_asym_ext.CCPAM.breakpoints.M  BreakpointsForDimension2=admireDB.aerodata_asym_ext.CCPAM.breakpoints.ALFA  BreakpointsForDimension3=[5, 7]  Table=admireDB.aerodata_asym_ext.CCPAM.newTable  ExtrapMethod=Clip  InternalRulePriority=Speed  RndMeth=Simplest  InputSameDT=on
      settings: InputPortMap=u0,u1
  Product2 : Product
  Ccp : Outport
  wires:
  mach_nd/1 -> CCPAM_ALFA_M/1
  CCPAM_ALFA_M/1 -> Product2/1
  Product2/1 -> Ccp/1
  pc/1 -> Product2/2
  angleOfAttack_deg/1 -> CCPAM_ALFA_M/2

== system ADMIRE/Aircraft/Aerodynamics/CentripetalForceCoefficient/MachRegion4/Ccr/Ccr_ ==
  mach_nd : Inport
  qacorr : Inport  Port=2
  rc : Inport  Port=3
  CCER_M_QA : Lookup_n-D  BreakpointsForDimension1=admireDB.aerodata_asym_ext.CCER.breakpoints.QA  BreakpointsForDimension2=admireDB.aerodata_asym_ext.CCER.breakpoints.M  BreakpointsForDimension3=[5, 7]  Table=admireDB.aerodata_asym_ext.CCER.newTable  ExtrapMethod=Clip  InternalRulePriority=Speed  RndMeth=Simplest  InputSameDT=on
      settings: InputPortMap=u0,u1
  CCRM_M : Lookup_n-D  NumberOfTableDimensions=1  BreakpointsForDimension1=admireDB.aerodata_asym_ext.CCRM.breakpoints.M  BreakpointsForDimension3=[5, 7]  Table=admireDB.aerodata_asym_ext.CCRM.newTable  ExtrapMethod=Clip  InternalRulePriority=Speed  RndMeth=Simplest  InputSameDT=on
  Product2 : Product  Inputs=3
  Ccr : Outport
  wires:
  CCER_M_QA/1 -> Product2/3
  qacorr/1 -> CCER_M_QA/1
  rc/1 -> Product2/2
  mach_nd/1 -> CCRM_M/1, CCER_M_QA/2
  CCRM_M/1 -> Product2/1
  Product2/1 -> Ccr/1

== system ADMIRE/Aircraft/Aerodynamics/NormalForceCoefficient/MachRegion2/Cndei/Subsystem ==
  <dEI> : Inport
  <angleOfAttack_deg> : Inport  Port=2
  CNMDEA_ALFA_DE_M : Lookup_n-D  NumberOfTableDimensions=3  BreakpointsForDimension1=admireDB.aerodata_sym.CNMDEA.breakpoints.ALFA  BreakpointsForDimension2=admireDB.aerodata_sym.CNMDEA.breakpoints.DE  BreakpointsForDimension3=admireDB.aerodata_sym.CNMDEA.breakpoints.M  Table=admireDB.aerodata_sym.CNMDEA.newTable  ExtrapMethod=Clip  InternalRulePriority=Speed  RndMeth=Simplest  InputSameDT=on
      settings: InputPortMap=u0,u1,u2
  CNMDEA_ALFA_DE_M1 : Lookup_n-D  NumberOfTableDimensions=3  BreakpointsForDimension1=admireDB.aerodata_sym.CNMDEA.breakpoints.ALFA  BreakpointsForDimension2=admireDB.aerodata_sym.CNMDEA.breakpoints.DE  BreakpointsForDimension3=admireDB.aerodata_sym.CNMDEA.breakpoints.M  Table=admireDB.aerodata_sym.CNMDEA.newTable  ExtrapMethod=Clip  InternalRulePriority=Speed  RndMeth=Simplest  InputSameDT=on
      settings: InputPortMap=u0,u1,u2
  Constant1 : Constant  Value=0
  Sum1 : Sum  Inputs=|+-
  mach_nd_cnst : Constant  Value=0.5
  Out1 : Outport
  wires:
  Constant1/1 -> CNMDEA_ALFA_DE_M1/2
  <dEI>/1 -> CNMDEA_ALFA_DE_M/2
  CNMDEA_ALFA_DE_M/1 -> Sum1/1
  CNMDEA_ALFA_DE_M1/1 -> Sum1/2
  Sum1/1 -> Out1/1
  mach_nd_cnst/1 -> CNMDEA_ALFA_DE_M/3, CNMDEA_ALFA_DE_M1/3
  <angleOfAttack_deg>/1 -> CNMDEA_ALFA_DE_M/1, CNMDEA_ALFA_DE_M1/1

== system ADMIRE/Aircraft/Aerodynamics/NormalForceCoefficient/MachRegion2/Cndei/Subsystem1 ==
  <dEI> : Inport
  <angleOfAttack_deg> : Inport  Port=2
  CNDEAL_DE_ALFA : Lookup_n-D  BreakpointsForDimension1=admireDB.aerodata_sym.CNDEAL.breakpoints.ALFA  BreakpointsForDimension2=admireDB.aerodata_sym.CNDEAL.breakpoints.DE  BreakpointsForDimension3=[5, 7]  Table=admireDB.aerodata_sym.CNDEAL.newTable  ExtrapMethod=Clip  InternalRulePriority=Speed  RndMeth=Simplest  InputSameDT=on
      settings: InputPortMap=u0,u1
  CNDEAL_DE_ALFA1 : Lookup_n-D  BreakpointsForDimension1=admireDB.aerodata_sym.CNDEAL.breakpoints.ALFA  BreakpointsForDimension2=admireDB.aerodata_sym.CNDEAL.breakpoints.DE  BreakpointsForDimension3=[5, 7]  Table=admireDB.aerodata_sym.CNDEAL.newTable  ExtrapMethod=Clip  InternalRulePriority=Speed  RndMeth=Simplest  InputSameDT=on
      settings: InputPortMap=u0,u1
  Constant : Constant  Value=0
  Sum : Sum  Inputs=|+-
  Out1 : Outport
  wires:
  <dEI>/1 -> CNDEAL_DE_ALFA/2
  CNDEAL_DE_ALFA/1 -> Sum/1
  Constant/1 -> CNDEAL_DE_ALFA1/2
  CNDEAL_DE_ALFA1/1 -> Sum/2
  Sum/1 -> Out1/1
  <angleOfAttack_deg>/1 -> CNDEAL_DE_ALFA/1, CNDEAL_DE_ALFA1/1

== system ADMIRE/Aircraft/Aerodynamics/NormalForceCoefficient/MachRegion2/Cndey/Subsystem ==
  dEY : Inport
  <angleOfAttack_deg> : Inport  Port=2
  CNMDEA_ALFA_DE_M : Lookup_n-D  NumberOfTableDimensions=3  BreakpointsForDimension1=admireDB.aerodata_sym.CNMDEA.breakpoints.ALFA  BreakpointsForDimension2=admireDB.aerodata_sym.CNMDEA.breakpoints.DE  BreakpointsForDimension3=admireDB.aerodata_sym.CNMDEA.breakpoints.M  Table=admireDB.aerodata_sym.CNMDEA.newTable  ExtrapMethod=Clip  InternalRulePriority=Speed  RndMeth=Simplest  InputSameDT=on
      settings: InputPortMap=u0,u1,u2
  CNMDEA_ALFA_DE_M1 : Lookup_n-D  NumberOfTableDimensions=3  BreakpointsForDimension1=admireDB.aerodata_sym.CNMDEA.breakpoints.ALFA  BreakpointsForDimension2=admireDB.aerodata_sym.CNMDEA.breakpoints.DE  BreakpointsForDimension3=admireDB.aerodata_sym.CNMDEA.breakpoints.M  Table=admireDB.aerodata_sym.CNMDEA.newTable  ExtrapMethod=Clip  InternalRulePriority=Speed  RndMeth=Simplest  InputSameDT=on
      settings: InputPortMap=u0,u1,u2
  Constant1 : Constant  Value=0
  Sum1 : Sum  Inputs=|+-
  mach_nd_cnst : Constant  Value=0.5
  Out1 : Outport
  wires:
  <angleOfAttack_deg>/1 -> CNMDEA_ALFA_DE_M1/1, CNMDEA_ALFA_DE_M/1
  mach_nd_cnst/1 -> CNMDEA_ALFA_DE_M1/3, CNMDEA_ALFA_DE_M/3
  Sum1/1 -> Out1/1
  CNMDEA_ALFA_DE_M1/1 -> Sum1/2
  CNMDEA_ALFA_DE_M/1 -> Sum1/1
  dEY/1 -> CNMDEA_ALFA_DE_M/2
  Constant1/1 -> CNMDEA_ALFA_DE_M1/2

== system ADMIRE/Aircraft/Aerodynamics/NormalForceCoefficient/MachRegion2/Cndey/Subsystem1 ==
  dEY : Inport
  <angleOfAttack_deg> : Inport  Port=2
  CNDEAL_DE_ALFA : Lookup_n-D  BreakpointsForDimension1=admireDB.aerodata_sym.CNDEAL.breakpoints.ALFA  BreakpointsForDimension2=admireDB.aerodata_sym.CNDEAL.breakpoints.DE  BreakpointsForDimension3=[5, 7]  Table=admireDB.aerodata_sym.CNDEAL.newTable  ExtrapMethod=Clip  InternalRulePriority=Speed  RndMeth=Simplest  InputSameDT=on
      settings: InputPortMap=u0,u1
  CNDEAL_DE_ALFA1 : Lookup_n-D  BreakpointsForDimension1=admireDB.aerodata_sym.CNDEAL.breakpoints.ALFA  BreakpointsForDimension2=admireDB.aerodata_sym.CNDEAL.breakpoints.DE  BreakpointsForDimension3=[5, 7]  Table=admireDB.aerodata_sym.CNDEAL.newTable  ExtrapMethod=Clip  InternalRulePriority=Speed  RndMeth=Simplest  InputSameDT=on
      settings: InputPortMap=u0,u1
  Constant : Constant  Value=0
  Sum : Sum  Inputs=|+-
  Out1 : Outport
  wires:
  <angleOfAttack_deg>/1 -> CNDEAL_DE_ALFA/1, CNDEAL_DE_ALFA1/1
  Sum/1 -> Out1/1
  CNDEAL_DE_ALFA1/1 -> Sum/2
  Constant/1 -> CNDEAL_DE_ALFA1/2
  CNDEAL_DE_ALFA/1 -> Sum/1
  dEY/1 -> CNDEAL_DE_ALFA/2

== system ADMIRE/Aircraft/Aerodynamics/NormalForceCoefficient/MachRegion2/Cndn/Subsystem ==
  dN : Inport
  angleOfAttack_deg : Inport  Port=2
  tflow : Inport  Port=3
  CNDNAL_DN_ALFA : Lookup_n-D  BreakpointsForDimension1=admireDB.aerodata_sym.CNDNAL.breakpoints.ALFA  BreakpointsForDimension2=admireDB.aerodata_sym.CNDNAL.breakpoints.DN  BreakpointsForDimension3=[5, 7]  Table=admireDB.aerodata_sym.CNDNAL.newTable  ExtrapMethod=Clip  InternalRulePriority=Speed  RndMeth=Simplest  InputSameDT=on
      settings: InputPortMap=u0,u1
  Product1 : Product
  Out1 : Outport
  wires:
  dN/1 -> CNDNAL_DN_ALFA/2  "dN"
  tflow/1 -> Product1/2  "tflow"
  angleOfAttack_deg/1 -> CNDNAL_DN_ALFA/1  "angleOfAttack_deg"
  Product1/1 -> Out1/1
  CNDNAL_DN_ALFA/1 -> Product1/1

== system ADMIRE/Aircraft/Aerodynamics/NormalForceCoefficient/MachRegion2/Cndn/Subsystem1 ==
  <dN> : Inport
  <angleOfAttack_deg> : Inport  Port=2
  <tfhigh> : Inport  Port=3
  CNDNH_M_DN_ALFA : Lookup_n-D  NumberOfTableDimensions=3  BreakpointsForDimension1=admireDB.aerodata_sym.CNDNH.breakpoints.M  BreakpointsForDimension2=admireDB.aerodata_sym.CNDNH.breakpoints.DN  BreakpointsForDimension3=admireDB.aerodata_sym.CNDNH.breakpoints.ALFA  Table=admireDB.aerodata_sym.CNDNH.newTable  ExtrapMethod=Clip  InternalRulePriority=Speed  RndMeth=Simplest  InputSameDT=on
      settings: InputPortMap=u0,u1,u2
  Product1 : Product
  mach_nd_cnst : Constant  Value=0.5
  Out1 : Outport
  wires:
  <dN>/1 -> CNDNH_M_DN_ALFA/2
  <tfhigh>/1 -> Product1/2
  <angleOfAttack_deg>/1 -> CNDNH_M_DN_ALFA/3
  CNDNH_M_DN_ALFA/1 -> Product1/1
  mach_nd_cnst/1 -> CNDNH_M_DN_ALFA/1
  Product1/1 -> Out1/1

== system ADMIRE/Aircraft/Aerodynamics/NormalForceCoefficient/MachRegion2/Cnq/Subsystem ==
  <angleOfAttack_deg> : Inport
  <tflow> : Inport  Port=2
  <tfhigh> : Inport  Port=3
  Abs : Abs
  CNQAL_ALFA : Lookup_n-D  NumberOfTableDimensions=1  BreakpointsForDimension1=admireDB.aerodata_sym.CNQAL.breakpoints.ALFA  BreakpointsForDimension3=[5, 7]  Table=admireDB.aerodata_sym.CNQAL.newTable  ExtrapMethod=Clip  InternalRulePriority=Speed  RndMeth=Simplest  InputSameDT=on
  CNQAM_ALFA_M : Lookup_n-D  BreakpointsForDimension1=admireDB.aerodata_sym.CNQAM.breakpoints.M  BreakpointsForDimension2=admireDB.aerodata_sym.CNQAM.breakpoints.ALFA  BreakpointsForDimension3=[5, 7]  Table=admireDB.aerodata_sym.CNQAM.newTable  ExtrapMethod=Clip  InternalRulePriority=Speed  RndMeth=Simplest  InputSameDT=on
      settings: InputPortMap=u0,u1
  Product : Product
  Product1 : Product
  Sum : Sum  Inputs=|++
  mach_nd_cnst : Constant  Value=0.5
  Out1 : Outport
  wires:
  <tfhigh>/1 -> Product1/2
  <tflow>/1 -> Product/2
  Product/1 -> Sum/1
  Sum/1 -> Out1/1
  CNQAL_ALFA/1 -> Product/1
  mach_nd_cnst/1 -> CNQAM_ALFA_M/1
  <angleOfAttack_deg>/1 -> CNQAM_ALFA_M/2, Abs/1
  Abs/1 -> CNQAL_ALFA/1
  Product1/1 -> Sum/2
  CNQAM_ALFA_M/1 -> Product1/1

== system ADMIRE/Aircraft/Aerodynamics/NormalForceCoefficient/MachRegion3/Cndei/Subsystem ==
  <angleOfAttack_deg> : Inport
  <dEI> : Inport  Port=2
  <mach_nd> : Inport  Port=3
  <eieff> : Inport  Port=4
  CNMDEA_ALFA_DE_M : Lookup_n-D  NumberOfTableDimensions=3  BreakpointsForDimension1=admireDB.aerodata_sym.CNMDEA.breakpoints.ALFA  BreakpointsForDimension2=admireDB.aerodata_sym.CNMDEA.breakpoints.DE  BreakpointsForDimension3=admireDB.aerodata_sym.CNMDEA.breakpoints.M  Table=admireDB.aerodata_sym.CNMDEA.newTable  ExtrapMethod=Clip  InternalRulePriority=Speed  RndMeth=Simplest  InputSameDT=on
      settings: InputPortMap=u0,u1,u2
  CNMDEA_ALFA_DE_M1 : Lookup_n-D  NumberOfTableDimensions=3  BreakpointsForDimension1=admireDB.aerodata_sym.CNMDEA.breakpoints.ALFA  BreakpointsForDimension2=admireDB.aerodata_sym.CNMDEA.breakpoints.DE  BreakpointsForDimension3=admireDB.aerodata_sym.CNMDEA.breakpoints.M  Table=admireDB.aerodata_sym.CNMDEA.newTable  ExtrapMethod=Clip  InternalRulePriority=Speed  RndMeth=Simplest  InputSameDT=on
      settings: InputPortMap=u0,u1,u2
  Constant : Constant  Value=0
  Product : Product
  Sum : Sum  Inputs=|+-
  Out1 : Outport
  wires:
  <eieff>/1 -> Product/2
  Product/1 -> Out1/1
  CNMDEA_ALFA_DE_M/1 -> Sum/1
  Constant/1 -> CNMDEA_ALFA_DE_M1/2
  <mach_nd>/1 -> CNMDEA_ALFA_DE_M/3, CNMDEA_ALFA_DE_M1/3
  Sum/1 -> Product/1
  <dEI>/1 -> CNMDEA_ALFA_DE_M/2
  <angleOfAttack_deg>/1 -> CNMDEA_ALFA_DE_M/1, CNMDEA_ALFA_DE_M1/1
  CNMDEA_ALFA_DE_M1/1 -> Sum/2

== system ADMIRE/Aircraft/Aerodynamics/NormalForceCoefficient/MachRegion3/Cndey/Subsystem ==
  <angleOfAttack_deg> : Inport
  <dEI> : Inport  Port=2
  <mach_nd> : Inport  Port=3
  <eieff> : Inport  Port=4
  CNMDEA_ALFA_DE_M : Lookup_n-D  NumberOfTableDimensions=3  BreakpointsForDimension1=admireDB.aerodata_sym.CNMDEA.breakpoints.ALFA  BreakpointsForDimension2=admireDB.aerodata_sym.CNMDEA.breakpoints.DE  BreakpointsForDimension3=admireDB.aerodata_sym.CNMDEA.breakpoints.M  Table=admireDB.aerodata_sym.CNMDEA.newTable  ExtrapMethod=Clip  InternalRulePriority=Speed  RndMeth=Simplest  InputSameDT=on
      settings: InputPortMap=u0,u1,u2
  CNMDEA_ALFA_DE_M1 : Lookup_n-D  NumberOfTableDimensions=3  BreakpointsForDimension1=admireDB.aerodata_sym.CNMDEA.breakpoints.ALFA  BreakpointsForDimension2=admireDB.aerodata_sym.CNMDEA.breakpoints.DE  BreakpointsForDimension3=admireDB.aerodata_sym.CNMDEA.breakpoints.M  Table=admireDB.aerodata_sym.CNMDEA.newTable  ExtrapMethod=Clip  InternalRulePriority=Speed  RndMeth=Simplest  InputSameDT=on
      settings: InputPortMap=u0,u1,u2
  Constant : Constant  Value=0
  Product : Product
  Sum : Sum  Inputs=|+-
  Out1 : Outport
  wires:
  CNMDEA_ALFA_DE_M1/1 -> Sum/2
  <angleOfAttack_deg>/1 -> CNMDEA_ALFA_DE_M1/1, CNMDEA_ALFA_DE_M/1
  <dEI>/1 -> CNMDEA_ALFA_DE_M/2
  Sum/1 -> Product/1
  <mach_nd>/1 -> CNMDEA_ALFA_DE_M1/3, CNMDEA_ALFA_DE_M/3
  Constant/1 -> CNMDEA_ALFA_DE_M1/2
  CNMDEA_ALFA_DE_M/1 -> Sum/1
  Product/1 -> Out1/1
  <eieff>/1 -> Product/2

== system ADMIRE/Aircraft/Aerodynamics/PitchMomentCoefficient/MachRegion1/Cpmdei/Subsystem ==
  <dEI> : Inport
  <angleOfAttack_deg> : Inport  Port=2
  <eieff> : Inport  Port=3
  CPMDEAL_DE_ALFA1 : Lookup_n-D  BreakpointsForDimension1=admireDB.aerodata_sym.CPMDEAL.breakpoints.ALFA  BreakpointsForDimension2=admireDB.aerodata_sym.CPMDEAL.breakpoints.DE  BreakpointsForDimension3=[5, 7]  Table=admireDB.aerodata_sym.CPMDEAL.newTable  ExtrapMethod=Clip  InternalRulePriority=Speed  RndMeth=Simplest  InputSameDT=on
      settings: InputPortMap=u0,u1
  CPMDEAL_DE_ALFA2 : Lookup_n-D  BreakpointsForDimension1=admireDB.aerodata_sym.CPMDEAL.breakpoints.ALFA  BreakpointsForDimension2=admireDB.aerodata_sym.CPMDEAL.breakpoints.DE  BreakpointsForDimension3=[5, 7]  Table=admireDB.aerodata_sym.CPMDEAL.newTable  ExtrapMethod=Clip  InternalRulePriority=Speed  RndMeth=Simplest  InputSameDT=on
      settings: InputPortMap=u0,u1
  Constant : Constant  Value=0
  Product : Product
  Sum : Sum  Inputs=|+-
  Out1 : Outport
  wires:
  <dEI>/1 -> CPMDEAL_DE_ALFA1/2
  Product/1 -> Out1/1
  CPMDEAL_DE_ALFA1/1 -> Sum/1
  CPMDEAL_DE_ALFA2/1 -> Sum/2
  Sum/1 -> Product/1
  <angleOfAttack_deg>/1 -> CPMDEAL_DE_ALFA1/1, CPMDEAL_DE_ALFA2/1
  Constant/1 -> CPMDEAL_DE_ALFA2/2
  <eieff>/1 -> Product/2

== system ADMIRE/Aircraft/Aerodynamics/PitchMomentCoefficient/MachRegion1/Cpmdey/Subsystem ==
  dEY : Inport
  angleOfAttack_deg : Inport  Port=2
  eoeff : Inport  Port=3
  CPMDEAL_DE_ALFA1 : Lookup_n-D  BreakpointsForDimension1=admireDB.aerodata_sym.CPMDEAL.breakpoints.ALFA  BreakpointsForDimension2=admireDB.aerodata_sym.CPMDEAL.breakpoints.DE  BreakpointsForDimension3=[5, 7]  Table=admireDB.aerodata_sym.CPMDEAL.newTable  ExtrapMethod=Clip  InternalRulePriority=Speed  RndMeth=Simplest  InputSameDT=on
      settings: InputPortMap=u0,u1
  CPMDEAL_DE_ALFA2 : Lookup_n-D  BreakpointsForDimension1=admireDB.aerodata_sym.CPMDEAL.breakpoints.ALFA  BreakpointsForDimension2=admireDB.aerodata_sym.CPMDEAL.breakpoints.DE  BreakpointsForDimension3=[5, 7]  Table=admireDB.aerodata_sym.CPMDEAL.newTable  ExtrapMethod=Clip  InternalRulePriority=Speed  RndMeth=Simplest  InputSameDT=on
      settings: InputPortMap=u0,u1
  Constant : Constant  Value=0
  Product : Product
  Sum : Sum  Inputs=|+-
  Out1 : Outport
  wires:
  eoeff/1 -> Product/2
  Constant/1 -> CPMDEAL_DE_ALFA2/2
  angleOfAttack_deg/1 -> CPMDEAL_DE_ALFA2/1, CPMDEAL_DE_ALFA1/1
  Sum/1 -> Product/1
  CPMDEAL_DE_ALFA2/1 -> Sum/2
  CPMDEAL_DE_ALFA1/1 -> Sum/1
  Product/1 -> Out1/1
  dEY/1 -> CPMDEAL_DE_ALFA1/2

== system ADMIRE/Aircraft/Aerodynamics/PitchMomentCoefficient/MachRegion1/Cpmdle/Subsystem ==
  <angleOfAttack_deg> : Inport
  <dE> : Inport  Port=2
  <dN> : Inport  Port=3
  <lef_deg> : Inport  Port=4
  CPMDLAL_ALFA : Lookup_n-D  NumberOfTableDimensions=1  BreakpointsForDimension1=admireDB.aerodata_sym.CPMDLAL.breakpoints.ALFA  BreakpointsForDimension3=[5, 7]  Table=admireDB.aerodata_sym.CPMDLAL.newTable  ExtrapMethod=Clip  InternalRulePriority=Speed  RndMeth=Simplest  InputSameDT=on
  CPMDLDEA_DE_ALFA : Lookup_n-D  BreakpointsForDimension1=admireDB.aerodata_sym.CPMDLDEA.breakpoints.ALFA  BreakpointsForDimension2=admireDB.aerodata_sym.CPMDLDEA.breakpoints.DE  BreakpointsForDimension3=[5, 7]  Table=admireDB.aerodata_sym.CPMDLDEA.newTable  ExtrapMethod=Clip  InternalRulePriority=Speed  RndMeth=Simplest  InputSameDT=on
      settings: InputPortMap=u0,u1
  CPMDLDNA_DN_ALFA : Lookup_n-D  BreakpointsForDimension1=admireDB.aerodata_sym.CPMDLDNA.breakpoints.ALFA  BreakpointsForDimension2=admireDB.aerodata_sym.CPMDLDNA.breakpoints.DN  BreakpointsForDimension3=[5, 7]  Table=admireDB.aerodata_sym.CPMDLDNA.newTable  ExtrapMethod=Clip  InternalRulePriority=Speed  RndMeth=Simplest  InputSameDT=on
      settings: InputPortMap=u0,u1
  Constant : Constant  Value=1/27
  Product : Product  Inputs=3
  Sum : Sum  Inputs=+++
  Out1 : Outport
  wires:
  Constant/1 -> Product/3
  <lef_deg>/1 -> Product/2
  <dN>/1 -> CPMDLDNA_DN_ALFA/2
  Product/1 -> Out1/1
  CPMDLDEA_DE_ALFA/1 -> Sum/2
  <angleOfAttack_deg>/1 -> CPMDLDNA_DN_ALFA/1, CPMDLDEA_DE_ALFA/1, CPMDLAL_ALFA/1
  CPMDLAL_ALFA/1 -> Sum/1
  Sum/1 -> Product/1
  CPMDLDNA_DN_ALFA/1 -> Sum/3
  <dE>/1 -> CPMDLDEA_DE_ALFA/2
